simulink library "tqd"  (R2021b)
settings: Solver=VariableStepAuto  StartTime=0.0  StopTime=10.0  RelTol=1e-3
undefined symbols (not defined in the file or in its folder): ATQD_AccelLimitInRange_X_rpm, ATQD_AccelLimitInRange_Y_Nm, ATQD_AccelLimitOvrKi_X_Nm, ATQD_AccelLimitOvrKp_X_Nm, ATQD_BOSMapD_X_rpm, ATQD_BOSMapD_Y_pct, ATQD_BOSMapR_X_rpm, ATQD_BOSMapR_Y_pct, ATQD_HVBCurrSmooth_X_A, ATQD_LHMTqMapDLC_X_rpm, ATQD_LHMTqMapDLC_Y_pct, ATQD_LHMTqMapRLC_X_rpm, ATQD_LHMTqMapRLC_Y_pct, ATQD_NormalMapDLC_X_rpm, ATQD_NormalMapDLC_Y_pct, ATQD_NormalTqDecSR_X_rpm, ATQD_NormalTqDecSR_Y_Nm, ATQD_NormalTqIncSR_X_rpm, ATQD_NormalTqIncSR_Y_Nm, ATQD_OPDMapRLC_X_rpm, ATQD_OPDMapRLC_Y_pct, ATQD_RollRegTorReq_X_rpm, ATQD_RollRegTorReq_Y_enum, ATQD_VehSpdLimitInRange_X_rpm, ATQD_VehSpdLimitInRange_Y_Nm, ATQD_VehSpdLimitOvrKi_X_Nm, ATQD_VehSpdLimitOvrKp_X_Nm, EIGHT_INT, ENUM_BRAKEPEDAL_PRESSED, ENUM_BRAKEPEDAL_RELEASED, ENUM_COMBOKEY_DOWN, ENUM_COMBOKEY_M1, ENUM_COMBOKEY_M2, ENUM_COMBOKEY_NONE, ENUM_COMBOKEY_RKNEE, ENUM_COMBOKEY_STOPLV, ENUM_COMBOKEY_UP, ENUM_CP2VKNEEREQ_REQUEST, ENUM_CP2VNLVREQ_LEVEL1, ENUM_CP2VNLVREQ_LEVEL2, ENUM_CP2VNLVREQ_LOWER, ENUM_CP2VNLVREQ_STOPLV, ENUM_CP2VNLVREQ_UPPER, ENUM_CREEPIND_DISABLE, ENUM_CREEPIND_READY, ENUM_CREEPIND_RUNNING, ENUM_CREEPIND_WARNING, ENUM_DRIVELINERELEASE_RELEASE, ENUM_EBSTORQUERWQ_LIMIT, ENUM_EBSTORQUERWQ_TORQUE, ENUM_ECPVCUDRM_CONFORT, ENUM_ECPVCUDRM_ECO, ENUM_ECPVCUDRM_NORMAL, ENUM_ECPVCUDRM_NOTAVAILABLE, ENUM_EMTqModeDrvBrk_Accel, ENUM_EMTqModeDrvBrk_Brake, ENUM_EMTqModeDrvBrk_Coast, ENUM_ETC2ACTDRIVEDIR_BACKWARD, ENUM_ETC2ACTDRIVEDIR_FORWARD, ENUM_ETC2ACTDRIVEDIR_STILL ... (+341)
libraries: simulink x109, hcu_lib x67
(part 4 of 13)

== system tqd/TQD/Main/Available Torqeu Limitation ==
  BInpConvert_outputs : Inport
  BSCPIn_outputs : Inport  Port=2
  VTQD_CoorTqDemRr_Nm : Inport  Port=3
  Bus Selector : BusSelector  OutputSignals=VTQD_TqCMDUpLim_Nm,VTQD_TqCMDLowLim_Nm,VTQD_TrqCMDForveZero_flg
  Bus Selector1 : BusSelector  OutputSignals=VDMM_EBSRCIncorrect_flg,VDMM_DTCEBSRCIncorrect_flg
  Constant14 : Constant  Value=KTQD_EBSTqLimGain_c
  Constant15 : Constant  Value=ONE_INT
  Constant19 : Constant  Value=KTQD_MotoringTqDemN_Nm
  LiuZgSwitch1 : Switch  Criteria=u2 ~= 0  Threshold=0.5
      settings: AttributesFormatString=<%<Criteria>>
  LiuzgSwitch1 : Switch  Criteria=u2 ~= 0
      settings: AttributesFormatString=<%<Criteria>>
  OR5 : Logic  Operator=OR  AllPortsSameDT=off  OutDataTypeStr=boolean
  Product : Product
  Saturation Dynamic : simulink/Discontinuities/Saturation Dynamic  OutMin=[]  OutMax=[]  OutDataTypeStr=Inherit: Same as second input  OutDataType=fixdt(1, 16)  OutScaling=2^-10  DoSatur=off
  VTQD_AfterAvailableTqDemRr_Nm : Outport
  wires:
  [VTQD_AfterAvailableTqDemRr_Nm] -> VTQD_AfterAvailableTqDemRr_Nm/1
  Bus Selector/2 -> [VTQD_TqCMDLowLim_Nm]  "<VTQD_TqCMDLowLim_Nm>"
  Bus Selector/1 -> [VTQD_TqCMDUpLim_Nm]  "<VTQD_TqCMDUpLim_Nm>"
  BInpConvert_outputs/1 -> Bus Selector/1
  VTQD_CoorTqDemRr_Nm/1 -> [VTQD_CoorTqDemRr_Nm]
  [VTQD_CoorTqDemRr_Nm] -> Saturation Dynamic/2
  [VTQD_TqCMDLowLim_Nm] -> Saturation Dynamic/3
  [VTQD_TqCMDUpLim_Nm] -> Saturation Dynamic/1
  LiuZgSwitch1/1 -> Product/2
  [VTQD_TrqCMDForveZero_flg] -> LiuzgSwitch1/2
  Constant15/1 -> LiuZgSwitch1/3
  Saturation Dynamic/1 -> Product/1
  OR5/1 -> LiuZgSwitch1/2
  Constant14/1 -> LiuZgSwitch1/1
  [VDMM_EBSRCIncorrect_flg] -> OR5/1
  LiuzgSwitch1/1 -> [VTQD_AfterAvailableTqDemRr_Nm]  "VTQD_AfterAvailableTqDemRr_Nm"
  Product/1 -> LiuzgSwitch1/3
  Constant19/1 -> LiuzgSwitch1/1
  [VDMM_DTCEBSRCIncorrect_flg] -> OR5/2
  Bus Selector/3 -> [VTQD_TrqCMDForveZero_flg]  "<VTQD_TrqCMDForveZero_flg>"
  BSCPIn_outputs/1 -> Bus Selector1/1
  Bus Selector1/1 -> [VDMM_EBSRCIncorrect_flg]  "<VDMM_EBSRCIncorrect_flg>"
  Bus Selector1/2 -> [VDMM_DTCEBSRCIncorrect_flg]  "<VDMM_DTCEBSRCIncorrect_flg>"

== system tqd/TQD/Main/Driver Torque Demmand ==
  BDCQ_InpConvert_outputs : Inport
  Bus Selector : BusSelector  OutputSignals=VTQD_EM1ReqTorqLimBrk_Nm,VTQD_EM1TorqueCtrlBrk_flg,VTQD_EM1ReqTorqLimDriv_Nm,VTQD_EM1TorqueCtrlDriv_flg,VTQD_RollRegTorReq_Nm,VTQD_RollingRegenEnable_flg,VTQD_PedalMapTq_Nm,VTQD_LostComTempBCU_flg,VTQD_BOSTqDecRate_pct
  Constant : Constant  Value=ONE_PERCENT
  KTQD_MCULostLimitTorq_gain : Gain  Gain=KTQD_MCULostLimitTorq_gain
  LiuZgSwitch12 : Switch  Criteria=u2 ~= 0  Threshold=0.5
      settings: AttributesFormatString=<%<Criteria>>
  LiuZgSwitch13 : Switch  Criteria=u2 ~= 0  Threshold=0.5
      settings: AttributesFormatString=<%<Criteria>>
  LiuZgSwitch14 : Switch  Criteria=u2 ~= 0  Threshold=0.5
      settings: AttributesFormatString=<%<Criteria>>
  Product : Product  Inputs=3
  Switch1 : Switch  Criteria=u2 ~= 0
      settings: AttributesFormatString=%<Criteria>
  VTQD_DriverTqDem_Nm : Outport
  wires:
  [VTQD_EM1TorqueCtrlDriv_flg] -> LiuZgSwitch12/2
  [VTQD_RollingRegenEnable_flg] -> LiuZgSwitch14/2
  LiuZgSwitch12/1 -> LiuZgSwitch13/3
  [VTQD_EM1TorqueCtrlBrk_flg] -> LiuZgSwitch13/2
  [VTQD_EM1ReqTorqLimBrk_Nm] -> LiuZgSwitch13/1
  [VTQD_EM1ReqTorqLimDriv_Nm] -> LiuZgSwitch12/1
  [VTQD_RollRegTorReq_Nm] -> LiuZgSwitch14/1
  LiuZgSwitch14/1 -> LiuZgSwitch12/3
  BDCQ_InpConvert_outputs/1 -> Bus Selector/1
  Bus Selector/1 -> [VTQD_EM1ReqTorqLimBrk_Nm]  "<VTQD_EM1ReqTorqLimBrk_Nm>"
  Bus Selector/2 -> [VTQD_EM1TorqueCtrlBrk_flg]  "<VTQD_EM1TorqueCtrlBrk_flg>"
  Bus Selector/3 -> [VTQD_EM1ReqTorqLimDriv_Nm]  "<VTQD_EM1ReqTorqLimDriv_Nm>"
  Bus Selector/4 -> [VTQD_EM1TorqueCtrlDriv_flg]  "<VTQD_EM1TorqueCtrlDriv_flg>"
  Bus Selector/5 -> [VTQD_RollRegTorReq_Nm]  "<VTQD_RollRegTorReq_Nm>"
  Bus Selector/6 -> [VTQD_RollingRegenEnable_flg]  "<VTQD_RollingRegenEnable_flg>"
  Bus Selector/7 -> [VTQD_PedalMapTq_Nm]  "<VTQD_PedalMapTq_Nm>"
  [VTQD_DriverTqDem_Nm] -> VTQD_DriverTqDem_Nm/1
  [VTQD_LostComTempBCU_flg] -> Switch1/2
  KTQD_MCULostLimitTorq_gain/1 -> Switch1/1
  Bus Selector/8 -> [VTQD_LostComTempBCU_flg]  "<VTQD_LostComTempBCU_flg>"
  LiuZgSwitch13/1 -> Switch1/3, KTQD_MCULostLimitTorq_gain/1
  Switch1/1 -> [VTQD_DriverTqDem_Nm]  "VTQD_DriverTqDem_Nm"
  Bus Selector/9 -> [VTQD_BOSTqDecRate_pct]  "<VTQD_BOSTqDecRate_pct>"
  Product/1 -> LiuZgSwitch14/3
  [VTQD_PedalMapTq_Nm] -> Product/1
  [VTQD_BOSTqDecRate_pct] -> Product/2
  Constant/1 -> Product/3

== system tqd/TQD/Main/Gear Ratio ==

== system tqd/TQD/Main/Motor Direction ==
  BInpConvert_outputs : Inport
  VTQD_TMTqReqRaw_Nm : Inport  Port=2
  AND : Logic  AllPortsSameDT=off  OutDataTypeStr=boolean
  Bus Selector : BusSelector  OutputSignals=VTQD_GearActualPosn_enum
  Constant1 : Constant  Value=ENUM_GEARACTUALPOSN_R
  Constant11 : Constant  Value=KTQD_AbsoluteMotorTqDir_flg
  Equal : RelationalOperator  Operator===  OutDataTypeStr=boolean  RndMeth=Simplest
  Gain : Gain  Gain=MINUSONE_FLOAT  OutDataTypeStr=single
  LiuZgSwitch8 : Switch  Criteria=u2 ~= 0  Threshold=0.5
      settings: AttributesFormatString=<%<Criteria>>
  VTQD_TMTqReq_Nm : Outport
  wires:
  VTQD_TMTqReqRaw_Nm/1 -> [VTQD_TMTqReqRaw_Nm]
  BInpConvert_outputs/1 -> Bus Selector/1
  Bus Selector/1 -> [VTQD_GearActualPosn_enum]  "<VTQD_GearActualPosn_enum>"
  [VTQD_TMTqReq_Nm] -> VTQD_TMTqReq_Nm/1
  Constant1/1 -> Equal/2
  AND/1 -> LiuZgSwitch8/2
  [VTQD_TMTqReqRaw_Nm] -> Gain/1
  Constant11/1 -> AND/1
  [VTQD_TMTqReqRaw_Nm] -> LiuZgSwitch8/3
  [VTQD_GearActualPosn_enum] -> Equal/1
  Gain/1 -> LiuZgSwitch8/1
  Equal/1 -> AND/2
  LiuZgSwitch8/1 -> [VTQD_TMTqReq_Nm]  "VTQD_TMTqReq_Nm"

== system tqd/TQD/Main/Ramp Input Torque ==
  BInpConvert_outputs : Inport
  BSCPIn_outputs : Inport  Port=2
  VTQD_AfterAvailableTqDemRr_Nm : Inport  Port=3
  Abs2 : Abs
  Bus Selector : BusSelector  OutputSignals=VTQD_VCUMCUCtrlMdTQD_enum
  Bus Selector1 : BusSelector  OutputSignals=task_time_s,VINP_MotorTrq_Nm
  Consant1 : Constant  Value=EPS
      settings: AttributesFormatString=%<Name>
  Consant2 : Constant  Value=KTQD_TorCtrlModeSwSmoTime_s  OutDataTypeStr=single
      settings: AttributesFormatString=%<Name>
  Consant3 : Constant  Value=KTQD_TorCtrlModeSwSmoTs_c  OutDataTypeStr=single
      settings: AttributesFormatString=%<Name>
  Constant3 : Constant  Value=ENUM_MCUCTRLMODE_SPEED
  Divide : Product  Inputs=*/
  Equal3 : RelationalOperator  Operator===  OutDataTypeStr=boolean  RndMeth=Simplest
  FirstOrderFilter3 : hcu_lib/Basic_Blocks/FirstOrderFilter
      settings: SourceProductName=HCU Relative Block Library
  Floor : Rounding
  Max : MinMax  Function=max  Inputs=2
  Resettable Delay : Delay  DelayLengthSource=Input port  DelayLength=1  DelayLengthUpperLimit=1000  InitialCondition=boolean(0)
      settings: AttributesFormatString=%<InitialCondition>  InputPortMap=u0,p1
  Switch1 : Switch  Criteria=u2 ~= 0
      settings: AttributesFormatString=%<Criteria>
  VTQD_RrRampInpTqRr_Nm : Outport
  wires:
  [VTQD_RrRampInpTqRr_Nm] -> VTQD_RrRampInpTqRr_Nm/1
  Bus Selector/1 -> [VTQD_VCUMCUCtrlMdTQD_enum]  "<VTQD_VCUMCUCtrlMdTQD_enum>"
  BInpConvert_outputs/1 -> Bus Selector/1
  VTQD_AfterAvailableTqDemRr_Nm/1 -> [VTQD_AfterAvailableTqDemRr_Nm]
  Floor/1 -> Resettable Delay/2
  [VTQD_AfterAvailableTqDemRr_Nm] -> Switch1/3
  Consant3/1 -> FirstOrderFilter3/3
  Constant3/1 -> Equal3/2
  [task_time_s] -> FirstOrderFilter3/2
  [VTQD_VCUMCUCtrlMdTQD_enum] -> Equal3/1
  Equal3/1 -> Resettable Delay/1
  FirstOrderFilter3/1 -> Switch1/1
  Consant2/1 -> Divide/1
  Resettable Delay/1 -> Switch1/2
  Divide/1 -> Floor/1
  [VINP_MotorTrq_Nm] -> Abs2/1
  Abs2/1 -> FirstOrderFilter3/1
  BSCPIn_outputs/1 -> Bus Selector1/1
  Bus Selector1/1 -> [task_time_s]  "<task_time_s>"
  Bus Selector1/2 -> [VINP_MotorTrq_Nm]  "<VINP_MotorTrq_Nm>"
  Max/1 -> Divide/2
  [task_time_s] -> Max/1
  Consant1/1 -> Max/2
  Switch1/1 -> [VTQD_RrRampInpTqRr_Nm]  "VTQD_RrRampInpTqRr_Nm"

== system tqd/TQD/Main/Torque Coordination ==
  BInpConvert_outputs : Inport
  VTQD_DriverTqDem_Nm : Inport  Port=2
  Bus Selector : BusSelector  OutputSignals=VTQD_GearActualPosn_enum
  Constant1 : Constant  Value=ENUM_GEARACTUALPOSN_R
  Constant2 : Constant  Value=ENUM_GEARACTUALPOSN_D
  Coordination Machine : Stateflow chart  TreatAsAtomicUnit=on
  Equal : RelationalOperator  Operator===  OutDataTypeStr=boolean  RndMeth=Simplest
  Equal1 : RelationalOperator  Operator===  OutDataTypeStr=boolean  RndMeth=Simplest
  NOT1 : Logic  Operator=NOT  AllPortsSameDT=off  OutDataTypeStr=boolean
  OR : Logic  Operator=OR  AllPortsSameDT=off  OutDataTypeStr=boolean
  VTQD_CoordTqDem_Nm : Outport
  wires:
  [VTQD_CoordTqDem_Nm] -> VTQD_CoordTqDem_Nm/1
  Bus Selector/1 -> [VTQD_GearActualPosn_enum]  "<VTQD_GearActualPosn_enum>"
  BInpConvert_outputs/1 -> Bus Selector/1
  [VTQD_GearActualPosn_enum] -> Equal/1
  Constant1/1 -> Equal/2
  Equal1/1 -> OR/1
  NOT1/1 -> [VTQD_NoSuitbleGear_flg]  "VTQD_NoSuitbleGear_flg"
  OR/1 -> NOT1/1
  Equal/1 -> OR/2
  Constant2/1 -> Equal1/2
  [VTQD_GearActualPosn_enum] -> Equal1/1
  VTQD_DriverTqDem_Nm/1 -> [VTQD_DriverTqDem_Nm]
  [VTQD_DriverTqDem_Nm] -> Coordination Machine/2(VTQD_DriverTqDem_Nm)
  [VTQD_NoSuitbleGear_flg] -> Coordination Machine/1(VTQD_NoSuitbleGear_flg)
  Coordination Machine/1(VTQD_CoordTqDem_Nm) -> [VTQD_CoordTqDem_Nm]

== system tqd/TQD/Main/Torque Distribution ==
  BInpConvert_outputs : Inport
  VTQD_CoordTqDem_Nm : Inport  Port=2
  Bus Selector : BusSelector  OutputSignals=VTQD_FrEDUSpRat_rat,VTQD_RrEDUSpRat_rat
  Product : Product
  Product1 : Product
  VTQD_CoorTqDemFr_Nm : Outport
  VTQD_CoorTqDemRr_Nm : Outport  Port=2
  wires:
  VTQD_CoordTqDem_Nm/1 -> [VTQD_CoordTqDem_Nm]
  BInpConvert_outputs/1 -> Bus Selector/1
  Bus Selector/1 -> [VTQD_FrEDUSpRat_rat]  "<VTQD_FrEDUSpRat_rat>"
  [VTQD_CoorTqDemFr_Nm] -> VTQD_CoorTqDemFr_Nm/1
  Bus Selector/2 -> [VTQD_RrEDUSpRat_rat]  "<VTQD_RrEDUSpRat_rat>"
  [VTQD_CoordTqDem_Nm] -> Product/1
  [VTQD_FrEDUSpRat_rat] -> Product/2
  Product/1 -> [VTQD_CoorTqDemFr_Nm]  "VTQD_CoorTqDemFr_Nm"
  [VTQD_RrEDUSpRat_rat] -> Product1/2
  [VTQD_CoordTqDem_Nm] -> Product1/1
  Product1/1 -> [VTQD_CoorTqDemRr_Nm]  "VTQD_CoorTqDemRr_Nm"
  [VTQD_CoorTqDemRr_Nm] -> VTQD_CoorTqDemRr_Nm/1

== system tqd/TQD/Main/Torque Ramp ==
  BInpConvert_outputs : Inport
  BSCPIn_outputs : Inport  Port=2
  VTQD_RrRampInpTqRr_Nm : Inport  Port=3
  Bus Selector : BusSelector  OutputSignals=VTQD_RampTs_c,VTQD_RampTqIncSR_Nm,VTQD_RampTqDecSR_Nm,VTQD_VCUMCUCtrlMdTQD_enum,VTQD_FinalTrqUpLim_Nm,VTQD_FinalTrqLowLim_Nm
  Bus Selector1 : BusSelector  OutputSignals=task_time_s
  Constant : Constant  Value=ZERO_FLOAT
  Constant6 : Constant  Value=ENUM_MCUCTRLMODE_TORQUE
  Constant7 : Constant  Value=ZERO_FLOAT
  Equal4 : RelationalOperator  Operator===  OutDataTypeStr=boolean  RndMeth=Simplest
  FirstOrderFilter1 : hcu_lib/Basic_Blocks/FirstOrderFilter
      settings: SourceProductName=HCU Relative Block Library
  Limit : hcu_lib/Basic_Blocks/Limit
      settings: SourceProductName=HCU Relative Block Library
  RateLimit1 : hcu_lib/Basic_Blocks/RateLimit
      settings: SourceProductName=HCU Relative Block Library
  Switch3 : Switch  Criteria=u2 ~= 0
      settings: AttributesFormatString=%<Criteria>
  Unit Delay3 : UnitDelay  InitialCondition=single(0)  SampleTime=-1
      settings: AttributesFormatString=%<InitialCondition>
  VTQD_TMTqReqRaw_Nm : Outport
  VTQD_RrRampTq_Nm : Outport  Port=2
  wires:
  [VTQD_TMTqReqRaw_Nm] -> VTQD_TMTqReqRaw_Nm/1
  Bus Selector/2 -> [VTQD_RampTqIncSR_Nm]  "<VTQD_RampTqIncSR_Nm>"
  Bus Selector/1 -> [VTQD_RampTs_c]  "<VTQD_RampTs_c>"
  BInpConvert_outputs/1 -> Bus Selector/1
  VTQD_RrRampInpTqRr_Nm/1 -> [VTQD_RrRampInpTqRr_Nm]
  Equal4/1 -> Switch3/2
  [VTQD_VCUMCUCtrlMdTQD_enum] -> Equal4/1
  Constant7/1 -> Switch3/3
  Constant6/1 -> Equal4/2
  Bus Selector1/1 -> [task_time_s]  "<task_time_s>"
  BSCPIn_outputs/1 -> Bus Selector1/1
  Bus Selector/3 -> [VTQD_RampTqDecSR_Nm]  "<VTQD_RampTqDecSR_Nm>"
  Bus Selector/4 -> [VTQD_VCUMCUCtrlMdTQD_enum]  "<VTQD_VCUMCUCtrlMdTQD_enum>"
  Bus Selector/5 -> [VTQD_FinalTrqUpLim_Nm]  "<VTQD_FinalTrqUpLim_Nm>"
  Bus Selector/6 -> [VTQD_FinalTrqLowLim_Nm]  "<VTQD_FinalTrqLowLim_Nm>"
  [VTQD_RrRampInpTqRr_Nm] -> FirstOrderFilter1/1
  [task_time_s] -> FirstOrderFilter1/2
  [VTQD_RampTs_c] -> FirstOrderFilter1/3
  FirstOrderFilter1/1 -> RateLimit1/1  "VTQD_TMTqReqSmooth_Nm"
  Constant/1 -> RateLimit1/2
  [task_time_s] -> RateLimit1/3
  [VTQD_RampTqIncSR_Nm] -> RateLimit1/4
  [VTQD_RampTqDecSR_Nm] -> RateLimit1/5
  RateLimit1/1 -> Unit Delay3/1
  Switch3/1 -> Limit/1
  [VTQD_FinalTrqUpLim_Nm] -> Limit/2
  [VTQD_FinalTrqLowLim_Nm] -> Limit/3
  Limit/1 -> [VTQD_TMTqReqRaw_Nm]  "VTQD_TMTqReqRaw_Nm"
  Unit Delay3/1 -> [VTQD_RrRampTq_Nm], Switch3/1  "VTQD_RrRampTq_Nm"
  [VTQD_RrRampTq_Nm] -> VTQD_RrRampTq_Nm/1

== system tqd/TQD/OutpConvert/ABS_System_Enable ==
  BInpConvert_outputs : Inport
  Bus Selector : BusSelector  OutputSignals=VTQD_EVDriveReady_flg
  Data Type Conversion : DataTypeConversion  OutDataTypeStr=boolean
  VTQD_TqReductEnable_flg : Outport
  wires:
  Data Type Conversion/1 -> [VTQD_TqReductEnable_flg]  "VTQD_TqReductEnable_flg"
  BInpConvert_outputs/1 -> Bus Selector/1
  Bus Selector/1 -> [VTQD_EVDriveReady_flg]  "<VTQD_EVDriveReady_flg>"
  [VTQD_EVDriveReady_flg] -> Data Type Conversion/1
  [VTQD_TqReductEnable_flg] -> VTQD_TqReductEnable_flg/1

== system tqd/TQD/OutpConvert/ADAS_DriverWheelTqDem ==
  BInpConvert_outputs : Inport
  BSCPIn_outputs : Inport  Port=2
  Bus Selector : BusSelector  OutputSignals=VTQD_PedalMapTq_Nm
  Bus Selector1 : BusSelector  OutputSignals=VINP_MotorTrq_Nm
  Constant1 : Constant  Value=KTQD_GearRatio_rate
  Constant5 : Constant  Value=KTQD_GearRatio_rate
  Product : Product
  Product1 : Product
  VTQD_ADASDriverDemWhTq_Nm : Outport
  VTQD_RealWhTq_Nm : Outport  Port=2
  wires:
  Product1/1 -> [VTQD_RealWhTq_Nm]  "VTQD_RealWhTq_Nm"
  Product/1 -> [VTQD_ADASDriverDemWhTq_Nm]  "VTQD_ADASDriverDemWhTq_Nm"
  BInpConvert_outputs/1 -> Bus Selector/1
  Bus Selector/1 -> [VTQD_PedalMapTq_Nm]  "<VTQD_PedalMapTq_Nm>"
  [VTQD_PedalMapTq_Nm] -> Product/1
  Bus Selector1/1 -> [VINP_MotorTrq_Nm]  "<VINP_MotorTrq_Nm>"
  BSCPIn_outputs/1 -> Bus Selector1/1
  [VINP_MotorTrq_Nm] -> Product1/1
  Constant1/1 -> Product1/2
  Constant5/1 -> Product/2
  [VTQD_RealWhTq_Nm] -> VTQD_RealWhTq_Nm/1
  [VTQD_ADASDriverDemWhTq_Nm] -> VTQD_ADASDriverDemWhTq_Nm/1

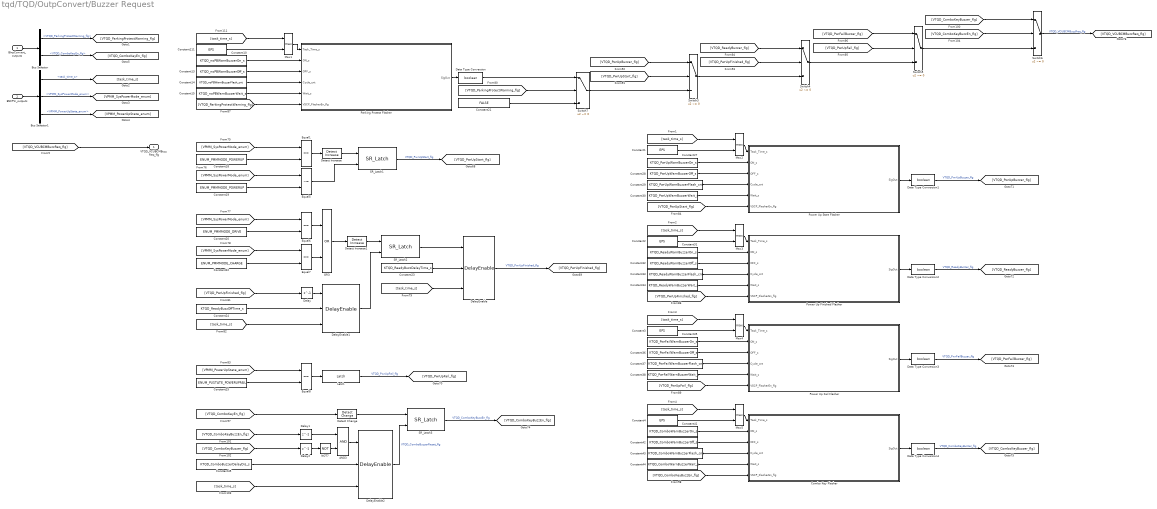
== system tqd/TQD/OutpConvert/Buzzer Request ==
  BInpConvert_outputs : Inport
  BSCPIn_outputs : Inport  Port=2
  AND3 : Logic  AllPortsSameDT=off  OutDataTypeStr=boolean
  Bus Selector : BusSelector  OutputSignals=VTQD_ParkingProtectWarning_flg,VTQD_ComboKeyEn_flg
  Bus Selector1 : BusSelector  OutputSignals=task_time_s,VPMM_SysPowerMode_enum,VPMM_PowerUpState_enum
  Combo Key Flasher : Subsystem
      settings: RTWSystemCode=Nonreusable function
  Constant{1..4,111} (5 alike) : Constant  Value=EPS
  Constant10 : Constant  Value=KTQD_noPBWarnBuzzerOn_s  VectorParams1D=off
  Constant13 : Constant  Value=KTQD_noPBWarnBuzzerOff_s  VectorParams1D=off
  Constant14 : Constant  Value=KTQD_noPBWarnBuzzerFlash_cnt  VectorParams1D=off
  Constant15 : Constant  Value=KTQD_noPBWarnBuzzerWait_s  VectorParams1D=off
  Constant18 : Constant  Value=ENUM_PMMMODE_POWERUP  VectorParams1D=off
  Constant19 : Constant  Value=ENUM_PMMMODE_POWERUP  VectorParams1D=off
  Constant20 : Constant  Value=ENUM_PMMMODE_DRIVE  VectorParams1D=off
  Constant21 : Constant  Value=FALSE  VectorParams1D=off
  Constant22 : Constant  Value=ENUM_PMMMODE_CHARGE  VectorParams1D=off
  Constant23 : Constant  Value=KTQD_ReadyBuzzDelayTime_s  VectorParams1D=off
  Constant24 : Constant  Value=KTQD_ReadyBuzzOffTime_s  VectorParams1D=off
  Constant25 : Constant  Value=ENUM_PUSTATE_POWERUPFAIL  VectorParams1D=off
  Constant27 : Constant  Value=KTQD_PwrUpWarnBuzzerOn_s  VectorParams1D=off
  Constant28 : Constant  Value=KTQD_PwrUpWarnBuzzerOff_s  VectorParams1D=off
  Constant29 : Constant  Value=KTQD_PwrUpWarnBuzzerFlash_cnt  VectorParams1D=off
  Constant30 : Constant  Value=KTQD_PwrUpWarnBuzzerWait_s  VectorParams1D=off
  Constant31 : Constant  Value=KTQD_ReadyWarnBuzzerOn_s  VectorParams1D=off
  Constant32 : Constant  Value=KTQD_ReadyWarnBuzzerOff_s  VectorParams1D=off
  Constant33 : Constant  Value=KTQD_ReadyWarnBuzzerFlash_cnt  VectorParams1D=off
  Constant34 : Constant  Value=KTQD_ReadyWarnBuzzerWait_s  VectorParams1D=off
  Constant35 : Constant  Value=KTQD_PwrFailWarnBuzzerOn_s  VectorParams1D=off
  Constant36 : Constant  Value=KTQD_PwrFailWarnBuzzerOff_s  VectorParams1D=off
  Constant37 : Constant  Value=KTQD_PwrFailWarnBuzzerFlash_cnt  VectorParams1D=off
  Constant38 : Constant  Value=KTQD_PwrFailWarnBuzzerWait_s  VectorParams1D=off
  Constant41 : Constant  Value=KTQD_ComboWarnBuzzerOn_s  VectorParams1D=off
  Constant42 : Constant  Value=KTQD_ComboWarnBuzzerOff_s  VectorParams1D=off
  Constant43 : Constant  Value=KTQD_ComboWarnBuzzerFlash_cnt  VectorParams1D=off
  Constant44 : Constant  Value=KTQD_ComboWarnBuzzerWait_s  VectorParams1D=off
  Constant45 : Constant  Value=KTQD_ComboBuzzerDelayDis_s  VectorParams1D=off
  Data Type Conversion{,1..4} (5 alike) : DataTypeConversion  OutDataTypeStr=boolean
  Delay : Delay  DelayLength=1  InitialCondition=boolean(0)
      settings: AttributesFormatString=%<InitialCondition>
  Delay1 : Delay  DelayLength=1  InitialCondition=boolean(0)
      settings: AttributesFormatString=%<InitialCondition>
  Delay2 : Delay  DelayLength=1  InitialCondition=boolean(0)
      settings: AttributesFormatString=%<InitialCondition>
  DelayEnable : hcu_lib/Basic_Blocks/DelayEnable
  DelayEnable1 : hcu_lib/Basic_Blocks/DelayEnable
  DelayEnable2 : hcu_lib/Basic_Blocks/DelayEnable
  Detect Change : simulink/Logic and Bit Operations/Detect Change  vinit=boolean(0)  OutDataTypeStr=boolean
  Detect Increase : simulink/Logic and Bit Operations/Detect Increase  vinit=boolean(0)  OutDataTypeStr=boolean
  Detect Increase1 : simulink/Logic and Bit Operations/Detect Increase  vinit=boolean(0)  OutDataTypeStr=boolean
  Equal{1,6..8} (4 alike) : RelationalOperator  Operator===  OutDataTypeStr=boolean  RndMeth=Simplest
  Equal5 : RelationalOperator  Operator=~=  OutDataTypeStr=boolean  RndMeth=Simplest
  Latch : hcu_lib/Basic_Blocks/Latch
  Max{1..5} (5 alike) : MinMax  Function=max  Inputs=2
  NOT7 : Logic  Operator=NOT  AllPortsSameDT=off  OutDataTypeStr=boolean
  OR3 : Logic  Operator=OR  AllPortsSameDT=off  OutDataTypeStr=boolean
  Parking Protect Flasher : Subsystem
      settings: RTWSystemCode=Nonreusable function
  Power Up Fail Flasher : Subsystem
      settings: RTWSystemCode=Nonreusable function
  Power Up Finished Flasher : Subsystem
      settings: RTWSystemCode=Nonreusable function
  Power Up Start Flasher : Subsystem
      settings: RTWSystemCode=Nonreusable function
  SR_Latch1 : hcu_lib/Basic_Blocks/SR_Latch
  SR_Latch2 : hcu_lib/Basic_Blocks/SR_Latch
  SR_Latch3 : hcu_lib/Basic_Blocks/SR_Latch
  Switch{3..7} (5 alike) : Switch  Criteria=u2 ~= 0
      settings: AttributesFormatString=%<Criteria>
  VTQD_VCUBCMBuzzReq_flg : Outport
  wires:
  Data Type Conversion4/1 -> [VTQD_ComboKeyBuzzer_flg]  "VTQD_ComboKeyBuzzer_flg"
  [VTQD_PwrUpFail_flg] -> Power Up Fail Flasher/6(VSCP_FlasherEn_flg)
  Switch4/1 -> Switch5/3
  [VTQD_PwrUpFinished_flg] -> Delay/1
  Constant23/1 -> DelayEnable/2
  Constant15/1 -> Parking Protect Flasher/5(Wait_s)
  Switch5/1 -> Switch6/3
  [VTQD_ReadyBuzzer_flg] -> Switch4/1
  Constant36/1 -> Power Up Fail Flasher/3(OFF_s)
  [VTQD_PwrUpFinished_flg] -> Switch4/2
  Power Up Finished Flasher/1(SigOut) -> Data Type Conversion2/1
  Latch/1 -> [VTQD_PwrUpFail_flg]  "VTQD_PwrUpFail_flg"
  DelayEnable/1 -> [VTQD_PwrUpFinished_flg]  "VTQD_PwrUpFinished_flg"
  Equal7/1 -> OR3/2
  Data Type Conversion/1 -> Switch7/1
  Switch7/1 -> Switch3/3
  Data Type Conversion3/1 -> [VTQD_PwrFailBuzzer_flg]  "VTQD_PwrFailBuzzer_flg"
  Equal1/1 -> Detect Increase/1
  Delay2/1 -> NOT7/1
  DelayEnable2/1 -> SR_Latch3/2  "VTQD_ComboBuzzerReset_flg"
  Constant35/1 -> Power Up Fail Flasher/2(ON_s)
  OR3/1 -> Detect Increase1/1
  Constant42/1 -> Combo Key Flasher/3(OFF_s)
  Constant45/1 -> DelayEnable2/2
  DelayEnable1/1 -> SR_Latch2/2
  Constant13/1 -> Parking Protect Flasher/3(OFF_s)
  Detect Increase/1 -> SR_Latch1/1
  Parking Protect Flasher/1(SigOut) -> Data Type Conversion/1
  [VTQD_ComboKeyEn_flg] -> Detect Change/1
  Delay1/1 -> AND3/1
  Constant38/1 -> Power Up Fail Flasher/5(Wait_s)
  [VTQD_ParkingProtectWarning_flg] -> Parking Protect Flasher/6(VSCP_FlasherEn_flg)
  Constant34/1 -> Power Up Finished Flasher/5(Wait_s)
  Constant25/1 -> Equal8/2
  Constant37/1 -> Power Up Fail Flasher/4(Cycle_cnt)
  [task_time_s] -> DelayEnable/3
  Equal6/1 -> OR3/1
  [VPMM_SysPowerMode_enum] -> Equal1/1
  Switch3/1 -> Switch4/3
  [VTQD_PwrUpFail_flg] -> Switch5/2
  [VTQD_ComboKeyBuzzer_flg] -> Delay2/1
  Constant21/1 -> Switch7/3
  Combo Key Flasher/1(SigOut) -> Data Type Conversion4/1
  Constant32/1 -> Power Up Finished Flasher/3(OFF_s)
  Equal8/1 -> Latch/1
  Constant14/1 -> Parking Protect Flasher/4(Cycle_cnt)
  Delay/1 -> DelayEnable1/1
  [task_time_s] -> DelayEnable1/3
  [VTQD_PwrUpBuzzer_flg] -> Switch3/1
  Power Up Start Flasher/1(SigOut) -> Data Type Conversion1/1
  Constant30/1 -> Power Up Start Flasher/5(Wait_s)
  [VTQD_ComboKeyBuzzEn_flg] -> Delay1/1
  AND3/1 -> DelayEnable2/1
  NOT7/1 -> AND3/2
  Constant41/1 -> Combo Key Flasher/2(ON_s)
  [VTQD_PwrUpFinished_flg] -> Power Up Finished Flasher/6(VSCP_FlasherEn_flg)
  Detect Change/1 -> SR_Latch3/1
  [VTQD_PwrFailBuzzer_flg] -> Switch5/1
  Power Up Fail Flasher/1(SigOut) -> Data Type Conversion3/1
  SR_Latch3/1 -> [VTQD_ComboKeyBuzzEn_flg]  "VTQD_ComboKeyBuzzEn_flg"
  Constant19/1 -> Equal5/2
  Constant18/1 -> Equal1/2
  [VTQD_ComboKeyBuzzEn_flg] -> Combo Key Flasher/6(VSCP_FlasherEn_flg)
  Constant43/1 -> Combo Key Flasher/4(Cycle_cnt)
  Constant24/1 -> DelayEnable1/2
  Data Type Conversion1/1 -> [VTQD_PwrUpBuzzer_flg]  "VTQD_PwrUpBuzzer_flg"
  [VTQD_PwrUpStart_flg] -> Switch3/2
  Equal5/1 -> SR_Latch1/2
  [VTQD_ComboKeyBuzzEn_flg] -> Switch6/2
  Constant31/1 -> Power Up Finished Flasher/2(ON_s)
  Data Type Conversion2/1 -> [VTQD_ReadyBuzzer_flg]  "VTQD_ReadyBuzzer_flg"
  Constant44/1 -> Combo Key Flasher/5(Wait_s)
  Constant22/1 -> Equal7/2
  [task_time_s] -> DelayEnable2/3
  [VTQD_ParkingProtectWarning_flg] -> Switch7/2
  [VTQD_ComboKeyBuzzer_flg] -> Switch6/1
  Switch6/1 -> [VTQD_VCUBCMBuzzReq_flg]  "VTQD_VCUBCMBuzzReq_flg"
  SR_Latch2/1 -> DelayEnable/1
  Detect Increase1/1 -> SR_Latch2/1
  [VPMM_SysPowerMode_enum] -> Equal7/1
  SR_Latch1/1 -> [VTQD_PwrUpStart_flg]  "VTQD_PwrUpStart_flg"
  [VPMM_SysPowerMode_enum] -> Equal5/1
  [VPMM_SysPowerMode_enum] -> Equal6/1
  Constant28/1 -> Power Up Start Flasher/3(OFF_s)
  [VPMM_PowerUpState_enum] -> Equal8/1
  [VTQD_PwrUpStart_flg] -> Power Up Start Flasher/6(VSCP_FlasherEn_flg)
  Constant20/1 -> Equal6/2
  Constant27/1 -> Power Up Start Flasher/2(ON_s)
  Constant33/1 -> Power Up Finished Flasher/4(Cycle_cnt)
  Constant29/1 -> Power Up Start Flasher/4(Cycle_cnt)
  Constant10/1 -> Parking Protect Flasher/2(ON_s)
  [task_time_s] -> Max1/1
  Constant111/1 -> Max1/2
  Max1/1 -> Parking Protect Flasher/1(Task_Time_s)
  [task_time_s] -> Max2/1
  Constant1/1 -> Max2/2
  Max2/1 -> Power Up Start Flasher/1(Task_Time_s)
  [task_time_s] -> Max3/1
  Constant2/1 -> Max3/2
  Max3/1 -> Power Up Finished Flasher/1(Task_Time_s)
  [task_time_s] -> Max4/1
  Constant3/1 -> Max4/2
  Max4/1 -> Power Up Fail Flasher/1(Task_Time_s)
  [task_time_s] -> Max5/1
  Constant4/1 -> Max5/2
  Max5/1 -> Combo Key Flasher/1(Task_Time_s)
  BSCPIn_outputs/1 -> Bus Selector1/1
  BInpConvert_outputs/1 -> Bus Selector/1
  Bus Selector1/1 -> [task_time_s]  "<task_time_s>"
  Bus Selector/1 -> [VTQD_ParkingProtectWarning_flg]  "<VTQD_ParkingProtectWarning_flg>"
  [VTQD_VCUBCMBuzzReq_flg] -> VTQD_VCUBCMBuzzReq_flg/1
  Bus Selector1/2 -> [VPMM_SysPowerMode_enum]  "<VPMM_SysPowerMode_enum>"
  Bus Selector1/3 -> [VPMM_PowerUpState_enum]  "<VPMM_PowerUpState_enum>"
  Bus Selector/2 -> [VTQD_ComboKeyEn_flg]  "<VTQD_ComboKeyEn_flg>"

== system tqd/TQD/OutpConvert/EC1 SCP ==
  Constant62 : Constant  Value=KTQD_MCUMaxRefTorq_Nm
  Constant98 : Constant  Value=ZERO_FLOAT  OutDataTypeStr=single
  Data Type Conversion{6..18,27..30,44..45,107,124..125} (22 alike) : DataTypeConversion  OutDataTypeStr=single
  Data Type Conversion{108..112} (5 alike) : DataTypeConversion  OutDataTypeStr=uint8
  VTQD_EC1EMSpdIdleP1_rpm : Outport
  VTQD_EC1PercTorqIdleP1_pct : Outport  Port=2
  VTQD_EC1EMSpdIdleP2_rpm : Outport  Port=3
  VTQD_EC1PercTorqIdleP2_pct : Outport  Port=4
  VTQD_EC1EMSpdIdleP3_rpm : Outport  Port=5
  VTQD_EC1PercTorqIdleP3_pct : Outport  Port=6
  VTQD_EC1EMSpdIdleP4_rpm : Outport  Port=7
  VTQD_EC1PercTorqIdleP4_pct : Outport  Port=8
  VTQD_EC1PercTorqIdleP5_pct : Outport  Port=9
  VTQD_EC1EMSpdIdleP5_rpm : Outport  Port=10
  VTQD_EC1EMRefTorq_Nm : Outport  Port=11
  VTQD_EC1EMMaxMEngOvrSP7_rpm : Outport  Port=12
  VTQD_EC1EMMaxMOvrTmt_s : Outport  Port=13
  VTQD_EC1EMReqSpdCtrlLoLmt_rpm : Outport  Port=14
  VTQD_EC1EMReqSpdCtrlUpLmt_rpm : Outport  Port=15
  VTQD_EC1EMReqTrqCtrlLoLmt_pct : Outport  Port=16
  VTQD_EC1EMReqTrqCtrlUpLmt_pct : Outport  Port=17
  VTQD_EC1EMExtRSCtrlUpLmt_rpm : Outport  Port=18
  VTQD_EC1EMMomOfInertia_kgpm2 : Outport  Port=19
  VTQD_EC1EMDefTrqLmt_rpm : Outport  Port=20
  VTQD_EC1EMSupVarRTSC1MSG_cnt : Outport  Port=21
  VTQD_EC1EMSupTSC1CtrlPG1_cnt : Outport  Port=22
  VTQD_EC1EMSupTSC1CtrlPG2_cnt : Outport  Port=23
  VTQD_EC1EMSupTSC1CtrlPG3_cnt : Outport  Port=24
  VTQD_EC1EMSupTSC1CtrlPG4_cnt : Outport  Port=25
  VTQD_EC1EMSpdHdleP6_rpm : Outport  Port=26
  VTQD_EC1EMGainEndSpdGvn_gain : Outport  Port=27
  wires:
  [DefaultValue16b] -> Data Type Conversion27/1
  Data Type Conversion7/1 -> VTQD_EC1PercTorqIdleP1_pct/1  "VTQD_EC1PercTorqIdleP1_pct"
  Constant62/1 -> Data Type Conversion12/1
  [DefaultValue16b] -> Data Type Conversion17/1
  Data Type Conversion28/1 -> VTQD_EC1PercTorqIdleP3_pct/1  "VTQD_EC1PercTorqIdleP3_pct"
  Data Type Conversion17/1 -> VTQD_EC1EMExtRSCtrlUpLmt_rpm/1  "VTQD_EC1EMExtRSCtrlUpLmt_rpm"
  [DefaultValue16b] -> Data Type Conversion44/1
  Data Type Conversion109/1 -> VTQD_EC1EMSupTSC1CtrlPG1_cnt/1  "VTQD_EC1EMSupTSC1CtrlPG1_cnt"
  [DefaultValue16b] -> Data Type Conversion16/1
  Data Type Conversion13/1 -> VTQD_EC1EMReqSpdCtrlLoLmt_rpm/1  "VTQD_EC1EMReqSpdCtrlLoLmt_rpm"
  [DefaultValue16b] -> Data Type Conversion11/1
  [DefaultValue16b] -> Data Type Conversion6/1
  Data Type Conversion45/1 -> VTQD_EC1PercTorqIdleP5_pct/1  "VTQD_EC1PercTorqIdleP5_pct"
  Data Type Conversion30/1 -> VTQD_EC1PercTorqIdleP4_pct/1  "VTQD_EC1PercTorqIdleP4_pct"
  Data Type Conversion125/1 -> VTQD_EC1EMGainEndSpdGvn_gain/1  "VTQD_EC1EMGainEndSpdGvn_gain"
  [DefaultValue8b] -> Data Type Conversion109/1
  Data Type Conversion108/1 -> VTQD_EC1EMSupVarRTSC1MSG_cnt/1  "VTQD_EC1EMSupVarRTSC1MSG_cnt"
  [DefaultValue16b] -> Data Type Conversion124/1
  Data Type Conversion27/1 -> VTQD_EC1EMSpdIdleP3_rpm/1  "VTQD_EC1EMSpdIdleP3_rpm"
  Data Type Conversion111/1 -> VTQD_EC1EMSupTSC1CtrlPG3_cnt/1  "VTQD_EC1EMSupTSC1CtrlPG3_cnt"
  Data Type Conversion12/1 -> VTQD_EC1EMRefTorq_Nm/1  "VTQD_EC1EMRefTorq_Nm"
  [DefaultValue8b] -> Data Type Conversion112/1
  Data Type Conversion44/1 -> VTQD_EC1EMSpdIdleP5_rpm/1  "VTQD_EC1EMSpdIdleP5_rpm"
  [DefaultValue8b] -> Data Type Conversion111/1
  Data Type Conversion14/1 -> VTQD_EC1EMReqSpdCtrlUpLmt_rpm/1  "VTQD_EC1EMReqSpdCtrlUpLmt_rpm"
  Data Type Conversion9/1 -> VTQD_EC1PercTorqIdleP2_pct/1  "VTQD_EC1PercTorqIdleP2_pct"
  [OfsetDefaultValue] -> Data Type Conversion28/1
  [DefaultValue16b] -> Data Type Conversion8/1
  [DefaultValue16b] -> Data Type Conversion125/1
  [DefaultValue8b] -> Data Type Conversion108/1
  [DefaultValue16b] -> Data Type Conversion13/1
  [OfsetDefaultValue] -> Data Type Conversion107/1
  Data Type Conversion10/1 -> VTQD_EC1EMMaxMEngOvrSP7_rpm/1  "VTQD_EC1EMMaxMEngOvrSP7_rpm"
  [DefaultValue16b] -> Data Type Conversion18/1
  Data Type Conversion107/1 -> VTQD_EC1EMReqTrqCtrlUpLmt_pct/1  "VTQD_EC1EMReqTrqCtrlUpLmt_pct"
  [OfsetDefaultValue] -> Data Type Conversion45/1
  [DefaultValue16b] -> Data Type Conversion29/1
  [OfsetDefaultValue] -> Data Type Conversion7/1
  Data Type Conversion16/1 -> VTQD_EC1EMDefTrqLmt_rpm/1  "VTQD_EC1EMDefTrqLmt_rpm"
  Data Type Conversion124/1 -> VTQD_EC1EMSpdHdleP6_rpm/1  "VTQD_EC1EMSpdHdleP6_rpm"
  Data Type Conversion29/1 -> VTQD_EC1EMSpdIdleP4_rpm/1  "VTQD_EC1EMSpdIdleP4_rpm"
  [DefaultValue16b] -> Data Type Conversion10/1
  Data Type Conversion6/1 -> VTQD_EC1EMSpdIdleP1_rpm/1  "VTQD_EC1EMSpdIdleP1_rpm"
  Data Type Conversion112/1 -> VTQD_EC1EMSupTSC1CtrlPG4_cnt/1  "VTQD_EC1EMSupTSC1CtrlPG4_cnt"
  [DefaultValue16b] -> Data Type Conversion14/1
  Data Type Conversion8/1 -> VTQD_EC1EMSpdIdleP2_rpm/1  "VTQD_EC1EMSpdIdleP2_rpm"
  [DefaultValue8b] -> Data Type Conversion110/1
  [OfsetDefaultValue] -> Data Type Conversion9/1
  [OfsetDefaultValue] -> Data Type Conversion15/1
  [OfsetDefaultValue] -> Data Type Conversion30/1
  Data Type Conversion11/1 -> VTQD_EC1EMMaxMOvrTmt_s/1  "VTQD_EC1EMMaxMOvrTmt_s"
  Data Type Conversion110/1 -> VTQD_EC1EMSupTSC1CtrlPG2_cnt/1  "VTQD_EC1EMSupTSC1CtrlPG2_cnt"
  Data Type Conversion18/1 -> VTQD_EC1EMMomOfInertia_kgpm2/1  "VTQD_EC1EMMomOfInertia_kgpm2"
  Data Type Conversion15/1 -> VTQD_EC1EMReqTrqCtrlLoLmt_pct/1  "VTQD_EC1EMReqTrqCtrlLoLmt_pct"
  Constant98/1 -> [OfsetDefaultValue], [DefaultValue8b], [DefaultValue16b]

== system tqd/TQD/OutpConvert/EEC3 SCP ==
  BInpConvert_outputs : Inport
  Abs4 : Abs
  Bus Selector : BusSelector  OutputSignals=VTQD_RollingRegenEnable_flg,VTQD_RollRegTorReq_Nm
  Constant1 : Constant  Value=ZERO_FLOAT
  Constant124 : Constant  Value=hex2dec('7D')
  Constant139 : Constant  Value=KTQD_MCUMaxRefTorq_Nm
  Constant2 : Constant  Value=EPS  OutDataTypeStr=single
  Data Type Conversion100 : DataTypeConversion  OutDataTypeStr=single
  Data Type Conversion99 : DataTypeConversion  OutDataTypeStr=single
  Divide2 : Product  Inputs=*/
  Fix2 : Rounding  Operator=fix
  Gain1 : Gain  Gain=HUNDRED  OutDataTypeStr=single
  Max : MinMax  Function=max  Inputs=2
  Switch47 : Switch  Criteria=u2 ~= 0
      settings: AttributesFormatString=%<Criteria>
  VTQD_EEC3NFricPercTorq_pct : Outport
  VTQD_EEC3EMPressLoss_pct : Outport  Port=2
  wires:
  Constant124/1 -> Data Type Conversion100/1
  Data Type Conversion99/1 -> [VTQD_EEC3NFricPercTorq_pct]  "VTQD_EEC3NFricPercTorq_pct"
  [VTQD_RollRegTorReq_Nm] -> Switch47/1
  Abs4/1 -> Gain1/1
  Fix2/1 -> Data Type Conversion99/1
  [VTQD_RollingRegenEnable_flg] -> Switch47/2
  Switch47/1 -> Divide2/1
  Divide2/1 -> Abs4/1
  Gain1/1 -> Fix2/1
  Data Type Conversion100/1 -> [VTQD_EEC3EMPressLoss_pct]  "VTQD_EEC3EMPressLoss_pct"
  BInpConvert_outputs/1 -> Bus Selector/1
  Bus Selector/1 -> [VTQD_RollingRegenEnable_flg]  "<VTQD_RollingRegenEnable_flg>"
  Bus Selector/2 -> [VTQD_RollRegTorReq_Nm]  "<VTQD_RollRegTorReq_Nm>"
  Constant1/1 -> Switch47/3
  Constant139/1 -> Max/1
  Constant2/1 -> Max/2
  Max/1 -> Divide2/2
  [VTQD_EEC3NFricPercTorq_pct] -> VTQD_EEC3NFricPercTorq_pct/1
  [VTQD_EEC3EMPressLoss_pct] -> VTQD_EEC3EMPressLoss_pct/1

== system tqd/TQD/OutpConvert/EMRC1 SCP ==
  BInpConvert_outputs : Inport
  BSCPIn_outputs : Inport  Port=2
  AND : Logic  AllPortsSameDT=off  OutDataTypeStr=boolean
  Abs1 : Abs
  Bus Selector : BusSelector  OutputSignals=VTQD_TqSource_enum,VTQD_GearActualPosn_enum,VTQD_RollingRegenEnable_flg,VTQD_TMTqCapGen_Nm
  Bus Selector1 : BusSelector  OutputSignals=VDHP_ActAPSPosn_pct,VINP_MotorTrq_Nm,VINP_MotorSpd_rpm,VDMM_EBSRCIncorrect_flg,VDMM_DTCEBSRCIncorrect_flg
  Constant1 : Constant  Value=EPS  OutDataTypeStr=single
  Constant125 : Constant  Value=ZERO_FLOAT
  Constant126 : Constant  Value=ZERO_FLOAT
  Constant128 : Constant  Value=ENUM_EMTqModeDrvBrk_Coast
  Constant129 : Constant  Value=ENUM_EMTqModeDrvBrk_Brake
  Constant130 : Constant  Value=KTQD_MCUMaxRefTorq_Nm
  Constant141 : Constant  Value=ENUM_EMTqModeDrvBrk_Accel
  Constant142 : Constant  Value=ENUM_TQSOURCE_ESC
  Constant146 : Constant  Value=ENUM_GEARACTUALPOSN_R
  Constant2 : Constant  Value=MINUSONE_FLOAT
  Constant3 : Constant  Value=ONE_FLOAT
  Constant4 : Constant  Value=ZERO_FLOAT  OutDataTypeStr=Inherit: Inherit via back propagation
  Constant5 : Constant  Value=ZERO_FLOAT  OutDataTypeStr=Inherit: Inherit via back propagation
  Constant6 : Constant  Value=EPS  OutDataTypeStr=single
  Constant67 : Constant  Value=KTQD_EBSIncMaxRegLim_pct
  Constant69 : Constant  Value=KTQD_MCUMaxRefTorq_Nm
  Constant7 : Constant  Value=0x7D  OutDataTypeStr=single
  Constant8 : Constant  Value=0xFF  OutDataTypeStr=single
  Constant86 : Constant  Value=KTQD_EMTqModeAPSAct_pct
  Constant9 : Constant  Value=0xEF  OutDataTypeStr=single
  Data Type Conversion{,1,117,121..123} (6 alike) : DataTypeConversion  OutDataTypeStr=single
  Data Type Conversion116 : DataTypeConversion  OutDataTypeStr=uint8
  Data Type Conversion2 : DataTypeConversion  OutDataTypeStr=uint8
  Divide : Product  Inputs=*/*
  Divide1 : Product  Inputs=*/
  Equal10 : RelationalOperator  Operator=>  OutDataTypeStr=boolean  RndMeth=Simplest
  Equal17 : RelationalOperator  Operator=>  OutDataTypeStr=boolean  RndMeth=Simplest
  Equal18 : RelationalOperator  Operator=<  OutDataTypeStr=boolean  RndMeth=Simplest
  Equal19 : RelationalOperator  Operator===  OutDataTypeStr=boolean  RndMeth=Simplest
  Equal20 : RelationalOperator  Operator===  OutDataTypeStr=boolean  RndMeth=Simplest
  Fix : Rounding  Operator=fix
  Fix1 : Rounding  Operator=fix
  Gain2 : Gain  Gain=HUNDRED  OutDataTypeStr=single
  Gain3 : Gain  Gain=HUNDRED  OutDataTypeStr=single
  Max : MinMax  Function=max  Inputs=2
  Max1 : MinMax  Function=max  Inputs=2
  OR : Logic  Operator=OR  AllPortsSameDT=off  OutDataTypeStr=boolean
  OR15 : Logic  Operator=OR  AllPortsSameDT=off  OutDataTypeStr=boolean
  Switch{21,42,44..46} (5 alike) : Switch  Criteria=u2 ~= 0
      settings: AttributesFormatString=%<Criteria>
  VTQD_EMRC1EMTquModeDrvBrk_enum : Outport
  VTQD_EMRC1ActEMpTrq_pct : Outport  Port=2
  VTQD_EMRC1ActEMOutSftSpd_rpm : Outport  Port=3
  VTQD_EMRC1ActEMpTrqHrls_pct : Outport  Port=4
  VTQD_EMRC1ActMaxAvaEMRecpTrq_pct : Outport  Port=5
  VTQD_EMRC1DrvDemEMRtapTrq_pct : Outport  Port=6
  VTQD_EMRC1RetSelNonEng_pct : Outport  Port=7
  VTQD_EMRC1SACtrlDev_cnt : Outport  Port=8
  wires:
  [VTQD_EMRC1ActEMpTrq_pct] -> Equal17/1
  Constant125/1 -> Equal17/2
  Equal19/1 -> Switch42/2
  OR15/1 -> Switch44/2
  [VTQD_RollingRegenEnable_flg] -> Switch46/2
  Data Type Conversion123/1 -> [VTQD_EMRC1ActMaxAvaEMRecpTrq_pct]  "VTQD_EMRC1ActMaxAvaEMRecpTrq_pct"
  Fix1/1 -> Data Type Conversion123/1
  Constant2/1 -> Switch42/1
  Equal20/1 -> AND/2
  Fix/1 -> Switch46/3
  Constant141/1 -> Switch45/1
  Constant86/1 -> Equal10/2
  Constant4/1 -> Switch46/1
  Constant128/1 -> Switch45/3
  [VTQD_EMRC1ActEMpTrq_pct] -> Equal18/1
  Constant129/1 -> Switch21/1
  Switch45/1 -> Switch21/3
  Equal18/1 -> AND/1
  Divide1/1 -> Gain3/1
  AND/1 -> Switch21/2
  Constant67/1 -> Switch44/1
  Switch44/1 -> Fix1/1
  Divide/1 -> Gain2/1
  Constant126/1 -> Equal18/2
  Constant142/1 -> Equal20/2
  Switch21/1 -> Data Type Conversion116/1
  Gain2/1 -> Fix/1
  Switch46/1 -> Data Type Conversion121/1
  [VTQD_TqSource_enum] -> Equal20/1
  OR/1 -> Switch45/2
  Constant5/1 -> Data Type Conversion117/1
  Data Type Conversion117/1 -> [VTQD_EMRC1ActEMpTrqHrls_pct]  "VTQD_EMRC1ActEMpTrqHrls_pct"
  Constant146/1 -> Equal19/2
  Equal17/1 -> OR/2
  Data Type Conversion116/1 -> [VTQD_EMRC1EMTquModeDrvBrk_enum]  "VTQD_EMRC1EMTquModeDrvBrk_enum"
  Abs1/1 -> Data Type Conversion122/1
  [VDHP_ActAPSPosn_pct] -> Equal10/1
  Data Type Conversion122/1 -> [VTQD_EMRC1ActEMOutSftSpd_rpm]  "VTQD_EMRC1ActEMOutSftSpd_rpm"
  Gain3/1 -> Switch44/3
  Data Type Conversion121/1 -> [VTQD_EMRC1ActEMpTrq_pct]  "VTQD_EMRC1ActEMpTrq_pct"
  Equal10/1 -> OR/1
  BInpConvert_outputs/1 -> Bus Selector/1
  Bus Selector/1 -> [VTQD_TqSource_enum]  "<VTQD_TqSource_enum>"
  Bus Selector1/1 -> [VDHP_ActAPSPosn_pct]  "<VDHP_ActAPSPosn_pct>"
  Bus Selector1/2 -> [VINP_MotorTrq_Nm]  "<VINP_MotorTrq_Nm>"
  BSCPIn_outputs/1 -> Bus Selector1/1
  [VTQD_EMRC1EMTquModeDrvBrk_enum] -> VTQD_EMRC1EMTquModeDrvBrk_enum/1
  [VTQD_GearActualPosn_enum] -> Equal19/1
  [VINP_MotorTrq_Nm] -> Divide/1
  Switch42/1 -> Divide/3
  Max/1 -> Divide/2
  Constant130/1 -> Max/1
  Constant1/1 -> Max/2
  Bus Selector/2 -> [VTQD_GearActualPosn_enum]  "<VTQD_GearActualPosn_enum>"
  Bus Selector/3 -> [VTQD_RollingRegenEnable_flg]  "<VTQD_RollingRegenEnable_flg>"
  Constant3/1 -> Switch42/3
  [VTQD_EMRC1ActEMpTrq_pct] -> VTQD_EMRC1ActEMpTrq_pct/1
  Bus Selector1/3 -> [VINP_MotorSpd_rpm]  "<VINP_MotorSpd_rpm>"
  [VINP_MotorSpd_rpm] -> Abs1/1
  [VTQD_EMRC1ActEMOutSftSpd_rpm] -> VTQD_EMRC1ActEMOutSftSpd_rpm/1
  [VTQD_EMRC1ActEMpTrqHrls_pct] -> VTQD_EMRC1ActEMpTrqHrls_pct/1
  Bus Selector1/4 -> [VDMM_EBSRCIncorrect_flg]  "<VDMM_EBSRCIncorrect_flg>"
  Bus Selector1/5 -> [VDMM_DTCEBSRCIncorrect_flg]  "<VDMM_DTCEBSRCIncorrect_flg>"
  [VTQD_TMTqCapGen_Nm] -> Divide1/1
  [VDMM_EBSRCIncorrect_flg] -> OR15/1
  [VDMM_DTCEBSRCIncorrect_flg] -> OR15/2
  Max1/1 -> Divide1/2
  Constant69/1 -> Max1/1
  Constant6/1 -> Max1/2
  [VTQD_EMRC1ActMaxAvaEMRecpTrq_pct] -> VTQD_EMRC1ActMaxAvaEMRecpTrq_pct/1
  Bus Selector/4 -> [VTQD_TMTqCapGen_Nm]  "<VTQD_TMTqCapGen_Nm>"
  [VTQD_EMRC1SACtrlDev_cnt] -> VTQD_EMRC1SACtrlDev_cnt/1
  [VTQD_EMRC1RetSelNonEng_pct] -> VTQD_EMRC1RetSelNonEng_pct/1
  [VTQD_EMRC1DrvDemEMRtapTrq_pct] -> VTQD_EMRC1DrvDemEMRtapTrq_pct/1
  Constant7/1 -> Data Type Conversion/1
  Constant8/1 -> Data Type Conversion1/1
  Data Type Conversion/1 -> [VTQD_EMRC1DrvDemEMRtapTrq_pct]  "VTQD_EMRC1DrvDemEMRtapTrq_pct"
  Data Type Conversion1/1 -> [VTQD_EMRC1RetSelNonEng_pct]  "VTQD_EMRC1RetSelNonEng_pct"
  Constant9/1 -> Data Type Conversion2/1
  Data Type Conversion2/1 -> [VTQD_EMRC1SACtrlDev_cnt]  "VTQD_EMRC1SACtrlDev_cnt"

== system tqd/TQD/OutpConvert/ETC1 SCP ==
  Constant61 : Constant  Value=ZERO_INT
  Data Type Conversion : DataTypeConversion  OutDataTypeStr=uint8
  VTQD_ETC1ShiftrPgs_enum : Outport
  wires:
  [VTQD_ETC1ShiftrPgs_enum] -> VTQD_ETC1ShiftrPgs_enum/1
  Data Type Conversion/1 -> [VTQD_ETC1ShiftrPgs_enum]  "VTQD_ETC1ShiftrPgs_enum"
  Constant61/1 -> Data Type Conversion/1

== system tqd/TQD/OutpConvert/ETC2 SCP ==
  BInpConvert_outputs : Inport
  Bus Selector : BusSelector  OutputSignals=VTQD_GearActualPosn_enum
  Constant75 : Constant  Value=ENUM_GEARACTUALPOSN_R
  Constant82 : Constant  Value=ENUM_GEARACTUALPOSN_D
  Constant83 : Constant  Value=ENUM_ETC2ACTDRIVEDIR_FORWARD
  Constant84 : Constant  Value=ENUM_ETC2ACTDRIVEDIR_STILL
  Constant85 : Constant  Value=ENUM_ETC2ACTDRIVEDIR_BACKWARD
  Equal11 : RelationalOperator  Operator===  OutDataTypeStr=boolean  RndMeth=Simplest
  Equal9 : RelationalOperator  Operator===  OutDataTypeStr=boolean  RndMeth=Simplest
  Switch22 : Switch  Criteria=u2 ~= 0
      settings: AttributesFormatString=%<Criteria>
  Switch23 : Switch  Criteria=u2 ~= 0
      settings: AttributesFormatString=%<Criteria>
  VTQD_ETC2ActDriveDirect_enum : Outport
  wires:
  Constant75/1 -> Equal11/2
  [VTQD_GearActualPosn_enum] -> Equal9/1
  [VTQD_GearActualPosn_enum] -> Equal11/1
  Equal9/1 -> Switch22/2
  Constant84/1 -> Switch23/3
  Constant82/1 -> Equal9/2
  Switch23/1 -> Switch22/3
  Constant83/1 -> Switch22/1
  Constant85/1 -> Switch23/1
  Switch22/1 -> [VTQD_ETC2ActDriveDirect_enum]  "VTQD_ETC2ActDriveDirect_enum"
  Equal11/1 -> Switch23/2
  [VTQD_ETC2ActDriveDirect_enum] -> VTQD_ETC2ActDriveDirect_enum/1
  Bus Selector/1 -> [VTQD_GearActualPosn_enum]  "<VTQD_GearActualPosn_enum>"
  BInpConvert_outputs/1 -> Bus Selector/1

== system tqd/TQD/OutpConvert/EVCU1 SCP ==
  note: EVCU1EMotorPerformance
  BInpConvert_outputs : Inport
  BSCPIn_outputs : Inport  Port=2
  AND1 : Logic  Inputs=3  AllPortsSameDT=off  OutDataTypeStr=boolean
  Abs : Abs
  Abs2 : Abs
  Abs3 : Abs
  Bus Selector : BusSelector  OutputSignals=VTQD_PedalMapTq_Nm,VTQD_GearActualPosn_enum
  Bus Selector1 : BusSelector  OutputSignals=VINP_MotorSpd_rpm,VINP_MotorTrq_Nm,VINP_B2VAvaPlsChgCurr_A,VINP_B2VSOC_pct,VINP_B2VFaultLv_enum
  Compare To Zero : simulink/Logic and Bit Operations/Compare To Zero  relop=>  OutDataTypeStr=boolean
  Compare To Zero1 : simulink/Logic and Bit Operations/Compare To Zero  relop=<  OutDataTypeStr=boolean
  Constant1 : Constant  Value=TWO_INT
  Constant123 : Constant  Value=KTQD_CurrEBrkAllow_A
  Constant150 : Constant  Value=ONE_INT
  Constant{3,94,151,186..187} (5 alike) : Constant  Value=ZERO_INT
  Constant155 : Constant  Value=KTQD_MCUMaxRefTorq_Nm
  Constant183 : Constant  Value=SIXTY
  Constant185 : Constant  Value=KTQD_SOCEBrkAllow_pct
  Constant188 : Constant  Value=ONE_INT
  Constant194 : Constant  Value=KTQD_RefMotorPower_kW
  Constant196 : Constant  Value=THOUSAND
  Constant197 : Constant  Value=ENUM_GEARACTUALPOSN_R
  Constant2 : Constant  Value=ONE_INT
  Constant4 : Constant  Value=EPS  OutDataTypeStr=single
  Constant5 : Constant  Value=EPS
  Constant6 : Constant  Value=PI
  Constant7 : Constant  Value=TWO
  Constant8 : Constant  Value=EPS  OutDataTypeStr=single
  Constant9 : Constant  Value=KTQD_RecuperHighSta_enum
  Data Type Conversion : DataTypeConversion  OutDataTypeStr=single
  Data Type Conversion{1,59,83,106} (4 alike) : DataTypeConversion  OutDataTypeStr=uint8
  Divide3 : Product  Inputs=*/
  Divide6 : Product  Inputs=*/
  Divide7 : Product  Inputs=*/
  Equal23 : RelationalOperator  Operator=>  OutDataTypeStr=boolean  RndMeth=Simplest
  Equal25 : RelationalOperator  Operator=<  OutDataTypeStr=boolean  RndMeth=Simplest
  Equal26 : RelationalOperator  Operator===  OutDataTypeStr=boolean  RndMeth=Simplest
  Equal33 : RelationalOperator  Operator===  OutDataTypeStr=boolean  RndMeth=Simplest
  Fix6 : Rounding  Operator=round
  Fix7 : Rounding  Operator=round
  Gain4 : Gain  Gain=HUNDRED  OutDataTypeStr=single
  Gain5 : Gain  Gain=HUNDRED  ParamDataTypeStr=single
  Gain9 : Gain  Gain=MINUSONE_FLOAT  OutDataTypeStr=single
  Max : MinMax  Function=max  Inputs=2
  Max1 : MinMax  Function=max  Inputs=2
  Max2 : MinMax  Function=max  Inputs=2
  Product2 : Product  Inputs=4
  Product6 : Product
  Relational Operator1 : RelationalOperator  OutDataTypeStr=boolean  RndMeth=Simplest
  Relay : Relay  OnSwitchValue=KTQD_VCUMCUDemHiPosVal_rpm + KTQD_MotorOverDev_rpm  OffSwitchValue=KTQD_VCUMCUDemHiPosVal_rpm  OnOutputValue=TRUE  OffOutputValue=FALSE
      settings: AttributesFormatString=|
      | ON:%<OnSwitchValue>
      | OFF:%<OffSwitchValue>
  Saturation14 : Saturate  UpperLimit=100000  LowerLimit=1
      settings: AttributesFormatString=|
      | UpperLimit: %<UpperLimit>
      | LowerLimit: %<LowerLimit>
  Switch{15,19,49,66,85..86} (6 alike) : Switch  Criteria=u2 ~= 0
      settings: AttributesFormatString=%<Criteria>
  VTQD_EVCU1ActDrvMode_enum : Outport
  VTQD_EVCU1WheelSlipdet_enum : Outport  Port=2
  VTQD_EVCU1EMotorSpd_rpm : Outport  Port=3
  VTQD_EVCU1EMotorOvrerSpd_enum : Outport  Port=4
  VTQD_EVCU1EMotorPerformance_pct : Outport  Port=5
  VTQD_EVCU1EBrakeTorqLow_enum : Outport  Port=6
  VTQD_EVCU1RecuperHighSta_enum : Outport  Port=7
  wires:
  [VTQD_EVCU1ActDrvMode_enum] -> VTQD_EVCU1ActDrvMode_enum/1
  Bus Selector/1 -> [VTQD_PedalMapTq_Nm]  "<VTQD_PedalMapTq_Nm>"
  BInpConvert_outputs/1 -> Bus Selector/1
  Relay/1 -> Switch49/2
  Switch19/1 -> Switch15/3
  Abs/1 -> Data Type Conversion/1
  Data Type Conversion59/1 -> [VTQD_EVCU1ActDrvMode_enum]  "VTQD_EVCU1ActDrvMode_enum"
  Switch15/1 -> Data Type Conversion59/1
  Compare To Zero/1 -> Switch15/2
  Constant94/1 -> Switch19/3
  Compare To Zero1/1 -> Switch19/2
  Constant151/1 -> Switch49/3
  Data Type Conversion106/1 -> [VTQD_EVCU1WheelSlipdet_enum]  "VTQD_EVCU1WheelSlipdet_enum"
  Switch49/1 -> [VTQD_EVCU1EMotorOvrerSpd_enum]  "VTQD_EVCU1EMotorOvrerSpd_enum"
  Constant150/1 -> Switch49/1
  Data Type Conversion/1 -> [VTQD_EVCU1EMotorSpd_rpm]  "VTQD_EVCU1EMotorSpd_rpm"
  [VTQD_PedalMapTq_Nm] -> Compare To Zero/1
  [VTQD_PedalMapTq_Nm] -> Compare To Zero1/1
  Constant1/1 -> Switch19/1
  Constant2/1 -> Switch15/1
  Constant3/1 -> Data Type Conversion106/1
  BSCPIn_outputs/1 -> Bus Selector1/1
  Bus Selector1/1 -> [VINP_MotorSpd_rpm]  "<VINP_MotorSpd_rpm>"
  [VINP_MotorSpd_rpm] -> Abs/1
  [VINP_MotorSpd_rpm] -> Relay/1
  Divide3/1 -> Gain5/1
  [VTQD_GearActualPosn_enum] -> Equal33/1
  Gain9/1 -> Switch85/1
  Divide6/1 -> Divide7/1
  Constant196/1 -> Product6/2
  [VINP_MotorTrq_Nm] -> Gain9/1
  Constant194/1 -> Product6/1
  Constant197/1 -> Equal33/2
  Divide7/1 -> Gain4/1
  [VINP_MotorSpd_rpm] -> Product2/1
  Constant155/1 -> Saturation14/1
  Product2/1 -> Divide6/1
  Switch85/1 -> Divide3/1
  Equal33/1 -> Switch85/2
  [VINP_MotorTrq_Nm] -> Switch85/3
  [VINP_MotorTrq_Nm] -> Product2/4
  Bus Selector1/2 -> [VINP_MotorTrq_Nm]  "<VINP_MotorTrq_Nm>"
  Constant6/1 -> Product2/2
  Gain5/1 -> [VTQD_EVCU1MotorTorque_pct]  "VTQD_EVCU1MotorTorque_pct"
  Gain4/1 -> [VTQD_EVCU1MotorPower_pct]  "VTQD_EVCU1MotorPower_pct"
  Constant7/1 -> Product2/3
  Max/1 -> Divide6/2
  Constant4/1 -> Max/2
  Constant183/1 -> Max/1
  Product6/1 -> Max1/1
  Constant5/1 -> Max1/2
  Max1/1 -> Divide7/2
  [VTQD_EVCU1MotorTorque_pct] -> Abs2/1
  [VTQD_EVCU1MotorTorque_pct] -> Switch86/3
  Abs3/1 -> Fix6/1
  Relational Operator1/1 -> Switch86/2
  Fix7/1 -> Relational Operator1/2
  Switch86/1 -> [VTQD_EVCU1EMotorPerformance_pct]  "VTQD_EVCU1EMotorPerformance_pct"
  Abs2/1 -> Fix7/1
  [VTQD_EVCU1MotorPower_pct] -> Switch86/1
  [VTQD_EVCU1MotorPower_pct] -> Abs3/1
  Fix6/1 -> Relational Operator1/1
  Bus Selector/2 -> [VTQD_GearActualPosn_enum]  "<VTQD_GearActualPosn_enum>"
  Constant8/1 -> Max2/2
  Saturation14/1 -> Max2/1
  Max2/1 -> Divide3/2
  Equal23/1 -> AND1/1
  Constant188/1 -> Switch66/3
  Constant186/1 -> Equal26/2
  [VINP_B2VFaultLv_enum] -> Equal26/1
  Equal26/1 -> AND1/3
  [VINP_B2VAvaPlsChgCurr_A] -> Equal23/1
  [VINP_B2VSOC_pct] -> Equal25/1
  Equal25/1 -> AND1/2
  Switch66/1 -> Data Type Conversion83/1
  AND1/1 -> Switch66/2
  Constant185/1 -> Equal25/2
  Constant187/1 -> Switch66/1
  Data Type Conversion83/1 -> [VTQD_EVCU1EBrakeTorqLow_enum]  "VTQD_EVCU1EBrakeTorqLow_enum"
  Constant123/1 -> Equal23/2
  [VTQD_EVCU1WheelSlipdet_enum] -> VTQD_EVCU1WheelSlipdet_enum/1
  [VTQD_EVCU1EMotorSpd_rpm] -> VTQD_EVCU1EMotorSpd_rpm/1
  [VTQD_EVCU1EMotorOvrerSpd_enum] -> VTQD_EVCU1EMotorOvrerSpd_enum/1
  [VTQD_EVCU1EMotorPerformance_pct] -> VTQD_EVCU1EMotorPerformance_pct/1
  [VTQD_EVCU1EBrakeTorqLow_enum] -> VTQD_EVCU1EBrakeTorqLow_enum/1
  Bus Selector1/3 -> [VINP_B2VAvaPlsChgCurr_A]  "<VINP_B2VAvaPlsChgCurr_A>"
  Bus Selector1/4 -> [VINP_B2VSOC_pct]  "<VINP_B2VSOC_pct>"
  Bus Selector1/5 -> [VINP_B2VFaultLv_enum]  "<VINP_B2VFaultLv_enum>"
  Constant9/1 -> Data Type Conversion1/1
  Data Type Conversion1/1 -> [VTQD_EVCU1RecuperHighSta_enum]  "VTQD_EVCU1RecuperHighSta_enum"
  [VTQD_EVCU1RecuperHighSta_enum] -> VTQD_EVCU1RecuperHighSta_enum/1
